simulink model "QuarcUDP"  (R2021a)
settings: Solver=FixedStepAuto  StartTime=0.0  StopTime=120  FixedStep=5e-3  RelTol=1e-3  EnableMultiTasking=on
libraries: quarc_library x1
settings Model: Creator=Navid  LastModifiedBy=Navid
settings SolverCC: PositivePriorityOrder=on
settings RTWCC: Description=QUARC Win64 Target Using Toolchain  SystemTargetFile=quarc_win64.tlc  Toolchain=QUARC win64 | nmake (64-bit Windows)  BuildConfiguration=Faster Runs
settings STFCustomTargetCC: TargetLangStandard=C99 (ISO)  ConcurrentExecutionCompliant=on  SystemTargetFile=quarc_win64.tlc
settings GRTTargetCC: ParMdlRefBuildCompliant=off  CompOptLevelCompliant=off  CombineOutputUpdateFcns=off  MatFileLogging=off  CPPClassGenCompliant=off  GRTInterface=on  ExtMode=on  ExtModeMexFile=quarc_comm

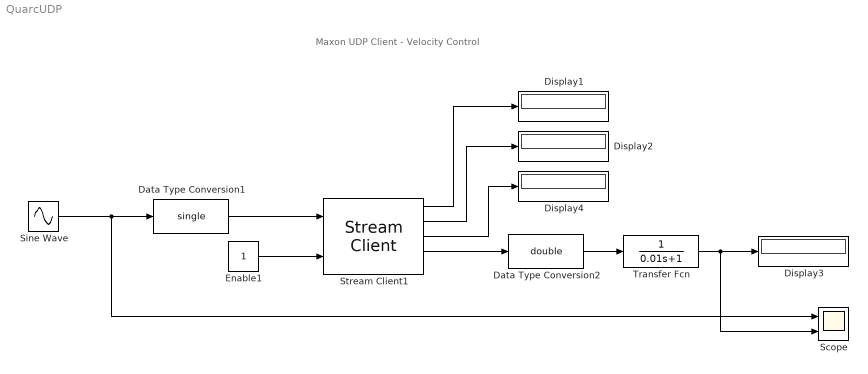
== system QuarcUDP ==
  note: Maxon UDP Client - Velocity Control
  Data Type Conversion1 : DataTypeConversion  OutDataTypeStr=single  RndMeth=Round  SaturateOnIntegerOverflow=on  LockScale=on
  Data Type Conversion2 : DataTypeConversion  OutDataTypeStr=double  RndMeth=Round  SaturateOnIntegerOverflow=on  LockScale=on
  Display{1..4} (4 alike) : Display
  Enable1 : Constant
  Scope : Scope  NumInputPorts=2
  Sine Wave : Sin  Amplitude=400  Frequency=2*pi*0.1  SampleTime=0
  Stream Client1 : quarc_library/Communications/Basic/Stream Client  uri_source=Specify via dialog (do not evaluate)  uri=udp://127.0.0.1:8888  apply_uri_to_all_configs=on  send_buffer_size=1024  receive_buffer_size=1024  byte_order=little endian (Intel - LSB first)  optimization=Minimum latency  send_options=Send most recent data  receive_options=Receive most recent data  default_value=[0]  sample_time=-1  active=on  implementation=Use blocking I/O in a separate thread  send_fifo_size=1000  receive_fifo_size=1000  send_priority=0  receive_priority=0  send_dimensions=off  receive_dimensions=off  max_dimensions=-1  data_type=single  type_expr=BusObject
      settings: AttributesFormatString="\"udp://127.0.0.1:8888\""
  Transfer Fcn : TransferFcn  Denominator=[0.01 1]
  wires:
  Stream Client1/1 -> Display1/1
  Stream Client1/3 -> Display4/1
  Enable1/1 -> Stream Client1/2
  Stream Client1/2 -> Display2/1
  Data Type Conversion1/1 -> Stream Client1/1
  Sine Wave/1 -> Scope/1, Data Type Conversion1/1
  Stream Client1/4 -> Data Type Conversion2/1
  Transfer Fcn/1 -> Scope/2, Display3/1
  Data Type Conversion2/1 -> Transfer Fcn/1
